simulink model "untitled"  (R2013a)
settings: Solver=ode45  StartTime=0.0  StopTime=10.0  RelTol=1e-3
libraries: aerolib6dof2 x1, aerolibschedule x1, aerolibutil x1, aerolibtransform2 x1
settings Model: Creator=victor  LastModifiedBy=victor

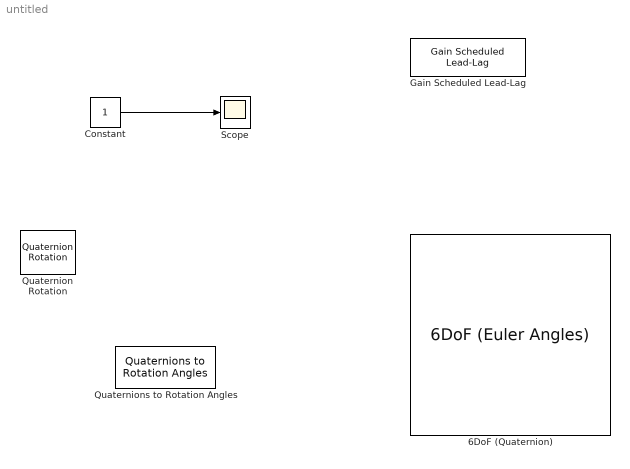
== system untitled ==
  6DoF (Quaternion) : aerolib6dof2/6DoF (Euler Angles)  units=Metric (MKS)  mtype=Fixed  rep=Quaternion  xme_0=[0 0 0]  Vm_0=w  eul_0=[0 0 0]  pm_0=[0 0 0]  mass_0=1.0  mass_e=0  mass_f=0  inertia=I  inertia_e=eye(3)  inertia_f=eye(3)  k_quat=1.0
  Constant : Constant
  Gain Scheduled Lead-Lag : aerolibschedule/Gain Scheduled Lead-Lag  x_initial=0
  Quaternion Rotation : aerolibutil/Quaternion Rotation
  Quaternions to Rotation Angles : aerolibtransform2/Quaternions to Rotation Angles  rotationOrder=ZXZ
  Scope : Scope
  wires:
  Constant/1 -> Scope/1
